simulink model "test_propagator"  (R2019b)
settings: Solver=ode15s  StartTime=0.0  StopTime=tf  RelTol=1e-3
InitFcn:
  | data
undefined symbols (not defined in the file): c_bo, inc, inertia, magnitude, n, omega_b, raan
libraries: simulink x4, blocklib x4
settings Model: SimulationMode=rapid-accelerator  Creator=Imanol  LastModifiedBy=imanol
settings ModelReferenceCC: ModelReferenceMinAlgLoopOccurrences=on
settings SFSimCC: CustomCodeUndefinedFunction=UseInterfaceOnly

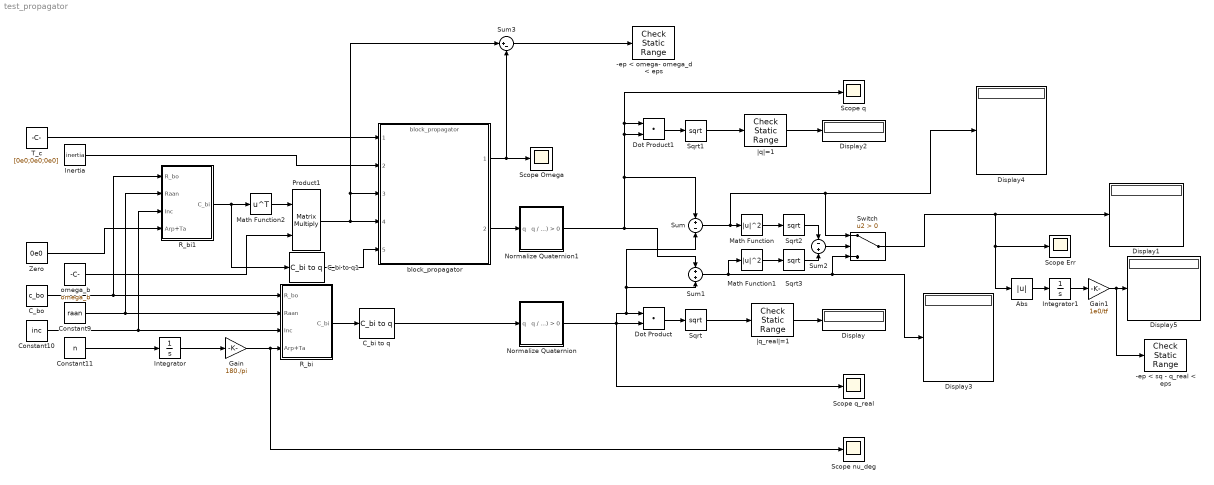
== system test_propagator ==
  -ep < omega- omega_d < eps : simulink/Model Verification/Check  Static Range  Description=- 1e-5 <= u <= 1e-5  max=1e-5  max_included=on  min=- 1e-5  min_included=on  enabled=on  stopWhenAssertionFail=on  export=off  icon=graphic
      settings: SourceProductName=Simulink  SourceProductBaseCode=SL
  -ep < sq - q_real < eps : simulink/Model Verification/Check  Static Range  Description=-1e-4 <= u <= 1e-4  max=1e-4  max_included=on  min=-1e-4  min_included=on  enabled=on  stopWhenAssertionFail=on  export=off  icon=graphic
      settings: SourceProductName=Simulink  SourceProductBaseCode=SL
  Abs : Abs
  C_bi to q : blocklib/C_bi to q  SystemSampleTime=-1  Latency=0  AutoFrameSizeCalculation=off
      settings: SourceProductName=Custom Library
  C_bi to q1 : blocklib/C_bi to q  SystemSampleTime=-1  Latency=0  AutoFrameSizeCalculation=off
      settings: SourceProductName=Custom Library
  C_bo : Constant  Value=c_bo
  Constant10 : Constant  Value=inc
  Constant11 : Constant  Value=n
  Constant9 : Constant  Value=raan
  Display{,1..5} (6 alike) : Display
      Display2 settings: Decimation=10000
  Dot Product : DotProduct  InputSameDT=on  OutDataTypeStr=Inherit: Inherit via internal rule
  Dot Product1 : DotProduct  InputSameDT=on  OutDataTypeStr=Inherit: Inherit via internal rule
  Gain : Gain  Gain=180./pi
  Gain1 : Gain  Gain=1e0/tf
  Inertia : Constant  Value=inertia
  Integrator : Integrator  InitialCondition=0e0
  Integrator1 : Integrator  InitialCondition=[0e0;0e0;0e0;0e0]
  Math Function : Math  Operator=magnitude^2  SignedPower=off  SaturateOnIntegerOverflow=on
  Math Function1 : Math  Operator=magnitude^2  SignedPower=off  SaturateOnIntegerOverflow=on
  Math Function2 : Math  Operator=transpose  SignedPower=off  SaturateOnIntegerOverflow=on
  Normalize Quaternion : Subsystem
  Normalize Quaternion1 : Subsystem
  Product1 : Product  Multiplication=Matrix(*)
  R_bi : Subsystem
  R_bi1 : Subsystem
  Scope Err : Scope
  Scope Omega : Scope
  Scope nu_deg : Scope
  Scope q : Scope
  Scope q_real : Scope
  Sqrt{,1..3} (4 alike) : Sqrt  SaturateOnIntegerOverflow=on
  Sum : Sum  Inputs=+|-
  Sum1 : Sum  Inputs=+|+
  Sum2 : Sum  Inputs=-|+
  Sum3 : Sum  Inputs=|+-
  Switch : Switch  Criteria=u2 > Threshold
  T_c : Constant  Value=[0e0;0e0;0e0]
  Zero : Constant  Value=0e0
  block_propagator : ModelReference  ModelNameDialog=block_propagator  SimulationMode=Normal  ModelReferenceVersion=1.37
  omega_b : Constant  Value=omega_b
  |q_real|=1 : simulink/Model Verification/Check  Static Range  Description=1e0 - 1e-5 <= u <= 1e0 + 1e-5  max=1e0 + 1e-5  max_included=on  min=1e0 - 1e-5  min_included=on  enabled=on  stopWhenAssertionFail=on  export=on  icon=graphic
      settings: SourceProductName=Simulink  SourceProductBaseCode=SL
  |q|=1 : simulink/Model Verification/Check  Static Range  Description=1e0 - 1e-4 <= u <= 1e0 + 1e-4  max=1e0 + 1e-4  max_included=on  min=1e0 - 1e-4  min_included=on  enabled=on  stopWhenAssertionFail=on  export=on  icon=graphic
      settings: SourceProductName=Simulink  SourceProductBaseCode=SL
  wires:
  T_c/1 -> block_propagator/1
  Inertia/1 -> block_propagator/2
  block_propagator/2 -> Normalize Quaternion1/1(q)
  block_propagator/1 -> Scope Omega/1, Sum3/2
  Dot Product/1 -> Sqrt/1
  Constant11/1 -> Integrator/1
  Dot Product1/1 -> Sqrt1/1
  Sqrt1/1 -> |q|=1/1
  Sqrt/1 -> |q_real|=1/1
  Sum/1 -> Math Function/1, Display4/1, Switch/1
  Integrator/1 -> Gain/1
  Constant9/1 -> R_bi1/2(Raan), R_bi/2(Raan)
  Constant10/1 -> R_bi1/3(Inc), R_bi/3(Inc)
  Gain/1 -> Scope nu_deg/1, R_bi/4(Arp+Ta)
  R_bi/1(C_bi) -> C_bi to q/1
  C_bo/1 -> R_bi1/1(R_bo), R_bi/1(R_bo)
  Zero/1 -> R_bi1/4(Arp+Ta)
  R_bi1/1(C_bi) -> Math Function2/1, C_bi to q1/1
  omega_b/1 -> Product1/2
  Product1/1 -> block_propagator/4, block_propagator/3, Sum3/1
  |q|=1/1 -> Display2/1
  |q_real|=1/1 -> Display/1
  C_bi to q1/1 -> block_propagator/5
  Normalize Quaternion/1(q / q(3) > 0) -> Scope q_real/1, Dot Product/1, Sum1/2, Sum/2, Dot Product/2
  C_bi to q/1 -> Normalize Quaternion/1(q)
  Normalize Quaternion1/1(q / q(3) > 0) -> Sum1/1, Scope q/1, Dot Product1/1, Dot Product1/2, Sum/1
  Sum1/1 -> Math Function1/1, Switch/3, Display3/1
  Switch/1 -> Display1/1, Scope Err/1, Abs/1
  Math Function/1 -> Sqrt2/1
  Sqrt2/1 -> Sum2/1
  Math Function1/1 -> Sqrt3/1
  Sqrt3/1 -> Sum2/2
  Sum2/1 -> Switch/2
  Sum3/1 -> -ep < omega- omega_d < eps/1
  Math Function2/1 -> Product1/1
  Integrator1/1 -> Gain1/1
  Gain1/1 -> -ep < sq - q_real < eps/1, Display5/1
  Abs/1 -> Integrator1/1

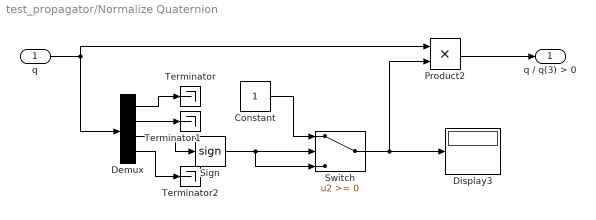
== system test_propagator/Normalize Quaternion ==
  q : Inport
  Constant : Constant
  Demux : Demux
  Display3 : Display
  Product2 : Product
  Sign : Signum
  Switch : Switch
  Terminator : Terminator
  Terminator1 : Terminator
  Terminator2 : Terminator
  q / q(3) > 0 : Outport
  wires:
  Demux/1 -> Terminator/1
  Demux/3 -> Sign/1
  q/1 -> Product2/1, Demux/1
  Product2/1 -> q / q(3) > 0/1
  Demux/4 -> Terminator2/1
  Sign/1 -> Switch/3, Switch/2
  Demux/2 -> Terminator1/1
  Constant/1 -> Switch/1
  Switch/1 -> Display3/1, Product2/2

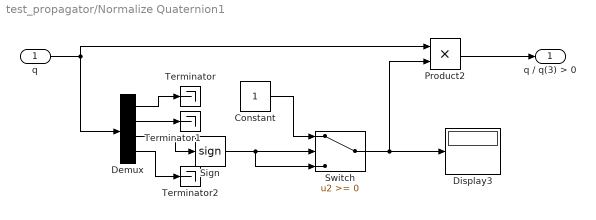
== system test_propagator/Normalize Quaternion1 ==
  q : Inport
  Constant : Constant
  Demux : Demux
  Display3 : Display
  Product2 : Product
  Sign : Signum
  Switch : Switch
  Terminator : Terminator
  Terminator1 : Terminator
  Terminator2 : Terminator
  q / q(3) > 0 : Outport
  wires:
  Demux/1 -> Terminator/1
  Demux/3 -> Sign/1
  q/1 -> Product2/1, Demux/1
  Product2/1 -> q / q(3) > 0/1
  Demux/4 -> Terminator2/1
  Sign/1 -> Switch/3, Switch/2
  Demux/2 -> Terminator1/1
  Constant/1 -> Switch/1
  Switch/1 -> Display3/1, Product2/2

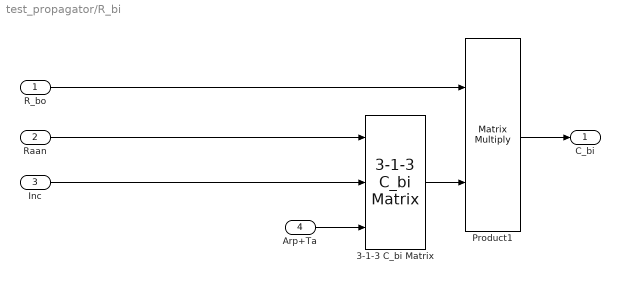
== system test_propagator/R_bi ==
  R_bo : Inport
  Raan : Inport  Port=2
  Inc : Inport  Port=3
  Arp+Ta : Inport  Port=4
  3-1-3 C_bi Matrix : blocklib/3-1-3 C_bi Matrix  SystemSampleTime=-1  Latency=0  AutoFrameSizeCalculation=off
      settings: SourceProductName=Custom Library
  Product1 : Product  Multiplication=Matrix(*)
  C_bi : Outport
  wires:
  Inc/1 -> 3-1-3 C_bi Matrix/2
  Product1/1 -> C_bi/1
  Raan/1 -> 3-1-3 C_bi Matrix/1
  3-1-3 C_bi Matrix/1 -> Product1/2
  R_bo/1 -> Product1/1
  Arp+Ta/1 -> 3-1-3 C_bi Matrix/3

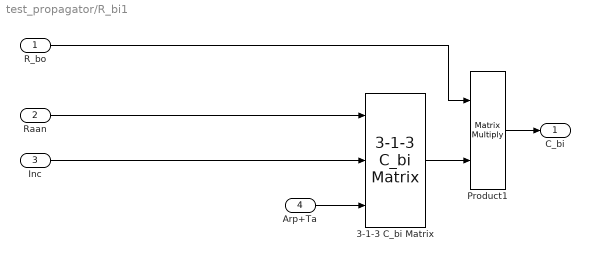
== system test_propagator/R_bi1 ==
  R_bo : Inport
  Raan : Inport  Port=2
  Inc : Inport  Port=3
  Arp+Ta : Inport  Port=4
  3-1-3 C_bi Matrix : blocklib/3-1-3 C_bi Matrix  SystemSampleTime=-1  Latency=0  AutoFrameSizeCalculation=off
      settings: SourceProductName=Custom Library
  Product1 : Product  Multiplication=Matrix(*)
  C_bi : Outport
  wires:
  Inc/1 -> 3-1-3 C_bi Matrix/2
  Product1/1 -> C_bi/1
  Raan/1 -> 3-1-3 C_bi Matrix/1
  3-1-3 C_bi Matrix/1 -> Product1/2
  R_bo/1 -> Product1/1
  Arp+Ta/1 -> 3-1-3 C_bi Matrix/3
